simulink model "Realised_inverter_EVOcargo"  (R2021b)
settings: Solver=ode23tb  StartTime=0.0  StopTime=0.02  MaxStep=2.5e-7  RelTol=1e-3  EnableMultiTasking=on
libraries: spsVoltageMeasurementLib x10, spsSeriesRLCBranchLib x9, spsCurrentMeasurementLib x8, spsMosfetLib x6, spsMeanLib x2, simulink x2, spsabctodq0Lib x2, slpidlib x1, spsIdealSwitchLib x1, spsPLL3phLib x1, spsThreePhaseBreakerLib x1, spsThreePhaseSourceLib x1
settings Model: SimulationMode=accelerator  Creator=Алексей  LastModifiedBy=nikol
settings SolverCC: ZeroCrossControl=DisableAll  ZeroCrossAlgorithm=Adaptive  AlgebraicLoopSolver=TrustRegion
settings DataIOCC: SaveFormat=Array  SaveOutput=off  SignalLogging=off  DSMLogging=off  SaveTime=off  ReturnWorkspaceOutputs=off
settings OptimizationCC: LifeSpan=inf
settings DebuggingCC: UnderspecifiedInitializationDetection=Classic  MergeDetectMultiDrivingBlocksExec=none  SolverPrmCheckMsg=warning  AllowSymbolicDim=off  SFUnexpectedBacktrackingDiag=warning  SFNoUnconditionalDefaultTransitionDiag=warning  SFExecutionAtInitializationDiag=none  SFMachineParentedDataDiag=warning  ArithmeticOperatorsInVariantConditions=warning
settings HardwareCC: ProdBitPerPointer=32  ProdBitPerSizeT=32  ProdBitPerPtrDiffT=32  ProdLargestAtomicFloat=None  ProdIntDivRoundTo=Undefined  ProdEndianess=Unspecified  ProdWordSize=32  ProdHWDeviceType=32-bit Generic
settings ModelReferenceCC: PropagateSignalLabelsOutOfModel=off
settings SFSimCC: SimUseLocalCustomCode=off  CustomCodeUndefinedFunction=UseInterfaceOnly
settings RTWCC: RTWUseLocalCustomCode=off
settings CodeAppCC: StateflowObjectComments=on
settings GRTTargetCC: TargetLangStandard=C89/C90 (ANSI)  RTWCAPISignals=on  RTWCAPIParams=on
settings ConfigComp: CovMetricSettings=dw  CovSaveCumulativeToWorkspaceVar=on  CovSaveSingleToWorkspaceVar=on  CovExternalEMLEnable=off  CovSFcnEnable=off
settings SimscapeCC: SimscapeNormalizeSystem=off

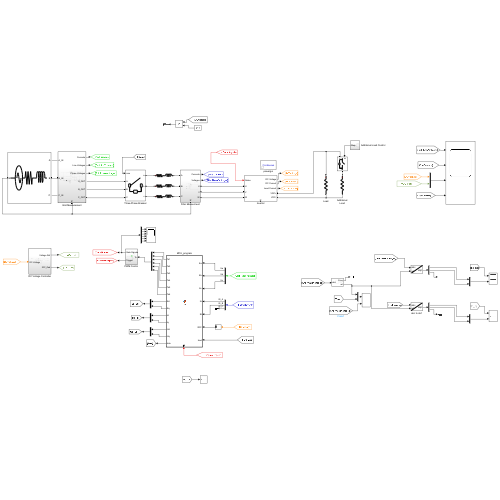
[thumbnail: Simulink's stored preview of the top-level diagram]
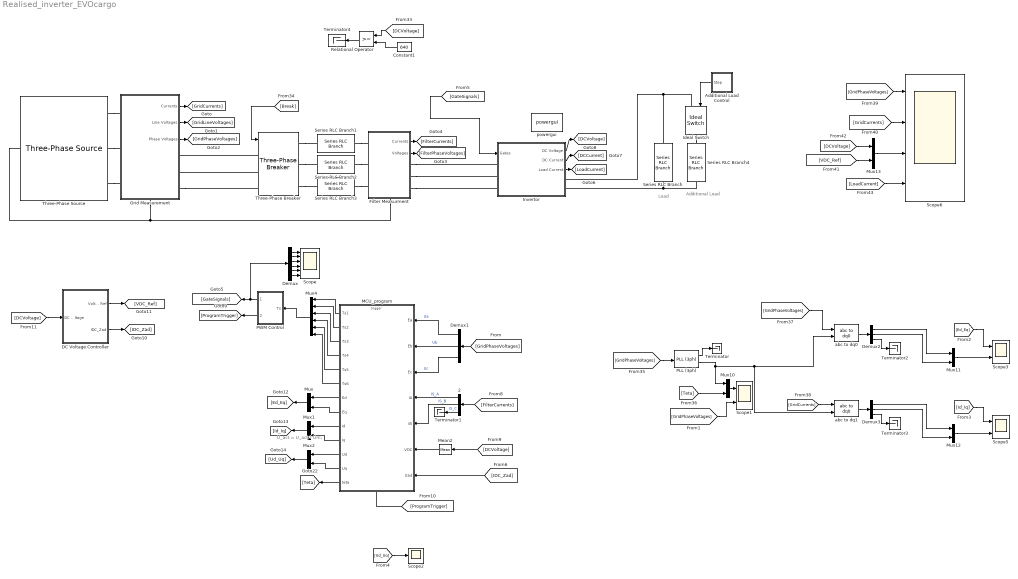
== system Realised_inverter_EVOcargo ==
  note: U_act = U_act * Um;
  note: Load
  note: Additional
      |     Load
  2 : Demux  Outputs=3
  Additional Load Control : Subsystem
  Constant1 : Constant  Value=640
  DC Voltage Controller : Subsystem
  Demux : Demux  Outputs=6
  Demux1 : Demux  Outputs=3
  Demux2 : Demux  Outputs=3
  Demux3 : Demux  Outputs=3
  Filter Measurment : Subsystem
      settings: PortSchema="{\"entries\":[{\"content\":{\"sides\":[{\"content\":{\"connectorIds\":[\"LConn1\",\"LConn2\",\"LConn3\"]},\"type\":\"ConnectorPlacement.EquallySpacedRectSide\",\"uuid\":\"07f1f610-fdaf-45a0-82ba-2fdf13164a36\"},{\"content\":{\"connectorIds\":[\"Out1\",\"Out2\",\"RConn1\",\"RConn2\",\"RConn3\"],\"side\":\"RIGHT\"},\"type\":\"ConnectorPlacement.EquallySpacedRectSide\",\"uuid\":\"0348acf2-7e1d-4672-a4d3-9caea07f27cd\"},{\"content\":{\"connectorIds\":[],\"side\":\"TOP\"},\"type\":\"ConnectorPlacement.EquallySpacedRectSide\",\"uuid\":\"be6f7439-4769-49ea-9688-befff8a6f50f\"},{\"content\":{\"connectorIds\":[\"RConn4\"],\"side\":\"BOTTOM\"},\"type\":\"ConnectorPlacement.EquallySpacedRectSide\",\"uuid\":\"239a5531-0ba1-4f36-bf56-c1872d73e635\"}]},\"type\":\"ConnectorPlacement.EquallySpacedConnector\",\"uuid\":\"325ea333-12da-4f70-8632-c5790302b8cd\"}],\"packageUris\":[\"http://schema.mathworks.com/mf0/Connector/R2020b\"],\"version\":\"1.0\"}"
  Grid Measurement : Subsystem
      settings: PortSchema="{\"entries\":[{\"content\":{\"sides\":[{\"content\":{\"connectorIds\":[\"LConn1\",\"LConn2\",\"LConn3\"]},\"type\":\"ConnectorPlacement.EquallySpacedRectSide\",\"uuid\":\"801c7675-c858-4350-92ae-14638809b1d2\"},{\"content\":{\"connectorIds\":[\"Out1\",\"Out2\",\"Out3\",\"RConn1\",\"RConn2\",\"RConn3\"],\"side\":\"RIGHT\"},\"type\":\"ConnectorPlacement.EquallySpacedRectSide\",\"uuid\":\"0a1e9bc1-9bed-4091-9780-772e4467681a\"},{\"content\":{\"connectorIds\":[],\"side\":\"TOP\"},\"type\":\"ConnectorPlacement.EquallySpacedRectSide\",\"uuid\":\"b82f9080-09d2-46b0-afde-a90803b4583a\"},{\"content\":{\"connectorIds\":[\"RConn4\"],\"side\":\"BOTTOM\"},\"type\":\"ConnectorPlacement.EquallySpacedRectSide\",\"uuid\":\"30cd731b-c919-4dce-85c5-af1a4330ad43\"}]},\"type\":\"ConnectorPlacement.EquallySpacedConnector\",\"uuid\":\"f4513950-4a40-4992-9ffd-40004173624b\"}],\"packageUris\":[\"http://schema.mathworks.com/mf0/Connector/R2020b\"],\"version\":\"1.0\"}"
  Ideal Switch : spsIdealSwitchLib/Ideal Switch  Ron=0.001  Lon=0  IC=0  Rs=1e5  Cs=inf  Measurements=off
  Invertor : Subsystem
      settings: PortSchema="{\"entries\":[{\"content\":{\"sides\":[{\"content\":{\"connectorIds\":[\"In1\",\"LConn1\",\"LConn2\",\"LConn3\"]},\"type\":\"ConnectorPlacement.EquallySpacedRectSide\",\"uuid\":\"92f6c0ba-483d-4b82-8aad-961a4c8cbef5\"},{\"content\":{\"connectorIds\":[\"Out1\",\"Out2\",\"Out3\",\"RConn1\",\"RConn2\"],\"side\":\"RIGHT\"},\"type\":\"ConnectorPlacement.EquallySpacedRectSide\",\"uuid\":\"ef3b9815-5c7f-4cd5-b6c4-990321a57132\"},{\"content\":{\"connectorIds\":[],\"side\":\"TOP\"},\"type\":\"ConnectorPlacement.EquallySpacedRectSide\",\"uuid\":\"4d71fcb3-3c6d-4f29-ac4d-ac71294aa9f2\"},{\"content\":{\"connectorIds\":[\"RConn3\"],\"side\":\"BOTTOM\"},\"type\":\"ConnectorPlacement.EquallySpacedRectSide\",\"uuid\":\"666ddd4c-3a12-4b0d-9e0a-750b3bb002db\"}]},\"type\":\"ConnectorPlacement.EquallySpacedConnector\",\"uuid\":\"7f816b13-2215-4e2c-95a7-fc33abc29cf3\"}],\"packageUris\":[\"http://schema.mathworks.com/mf0/Connector/R2020b\"],\"version\":\"1.0\"}"
  MCU_program : MATLAB Function  TreatAsAtomicUnit=on
  Mean2 : spsMeanLib/Mean  Freq=20000  Vinit=540  Ts=0
  Mux{,1..2,10..13} (7 alike) : Mux  Inputs=2
  Mux4 : Mux  Inputs=6
  PLL (3ph) : spsPLL3phLib/PLL (3ph)  Fmin=45  Par_Init=[0, 50]  ParK=[180, 3200, 1]  TcD=1e-4  MaxRateChangeFreq=12  FilterCutOffFreq=25  Ts=0  AGC=on
  PWM Control : Subsystem
      settings: PortSchema="{\"entries\":[{\"content\":{\"sides\":[{\"content\":{\"connectorIds\":[\"Out1\",\"Out2\"]},\"type\":\"ConnectorPlacement.EquallySpacedRectSide\",\"uuid\":\"d8b25c18-834a-4f60-b770-e16f9b0f8403\"},{\"content\":{\"connectorIds\":[\"In1\"],\"side\":\"RIGHT\"},\"type\":\"ConnectorPlacement.EquallySpacedRectSide\",\"uuid\":\"9dff51bf-dc9f-458e-a11e-8fbf0558d32b\"},{\"content\":{\"connectorIds\":[],\"side\":\"TOP\"},\"type\":\"ConnectorPlacement.EquallySpacedRectSide\",\"uuid\":\"abed77ec-c94b-4080-8d8e-77a9694eba29\"}]},\"type\":\"ConnectorPlacement.EquallySpacedConnector\",\"uuid\":\"310198e6-a417-4af9-8ce6-7d116e9fc291\"}],\"packageUris\":[\"http://schema.mathworks.com/mf0/Connector/R2020b\"],\"version\":\"1.0\"}"
  Relational Operator : RelationalOperator  OutDataTypeStr=boolean  RndMeth=Simplest
  Scope : Scope  NumInputPorts=6
  Scope1 : Scope  NumInputPorts=2
  Scope2 : Scope
  Scope3 : Scope  NumInputPorts=2
  Scope5 : Scope  NumInputPorts=2
  Scope6 : Scope  NumInputPorts=4
  Series RLC Branch : spsSeriesRLCBranchLib/Series RLC Branch  LConnTagsString=__new0  RConnTagsString=__new0  BranchType=R  Resistance=25  Inductance=1e-3  SetiL0=off  InitialCurrent=0  Capacitance=1e-6  Setx0=off  InitialVoltage=0  Measurements=None
  Series RLC Branch1 : spsSeriesRLCBranchLib/Series RLC Branch  LConnTagsString=__new0  RConnTagsString=__new0  BranchType=RL  Resistance=1e-3  Inductance=200e-6  SetiL0=off  InitialCurrent=0  Capacitance=1e-6  Setx0=off  InitialVoltage=0  Measurements=None
  Series RLC Branch2 : spsSeriesRLCBranchLib/Series RLC Branch  LConnTagsString=__new0  RConnTagsString=__new0  BranchType=RL  Resistance=1e-3  Inductance=200e-6  SetiL0=off  InitialCurrent=0  Capacitance=1e-6  Setx0=off  InitialVoltage=0  Measurements=None
  Series RLC Branch3 : spsSeriesRLCBranchLib/Series RLC Branch  LConnTagsString=__new0  RConnTagsString=__new0  BranchType=RL  Resistance=1e-3  Inductance=200e-6  SetiL0=off  InitialCurrent=0  Capacitance=1e-6  Setx0=off  InitialVoltage=0  Measurements=None
  Series RLC Branch4 : spsSeriesRLCBranchLib/Series RLC Branch  LConnTagsString=__new0  RConnTagsString=__new0  BranchType=R  Resistance=25  Inductance=1e-3  SetiL0=off  InitialCurrent=0  Capacitance=1e-6  Setx0=off  InitialVoltage=0  Measurements=None
  Terminator{,1..4} (5 alike) : Terminator
  Three-Phase Breaker : spsThreePhaseBreakerLib/Three-Phase Breaker  InitialState=open  SwitchA=on  SwitchB=on  SwitchC=on  SwitchTimes="[1/60  5/60]"  External=on  BreakerResistance=0.01  SnubberResistance=0.01  SnubberCapacitance=inf  Measurements=None
  Three-Phase Source : spsThreePhaseSourceLib/Three-Phase Source  InternalConnection=Yn  VoltagePhases=on  Voltage=200  PhaseAngle=0  Voltage_phases=[220 220 220]  PhaseAngles_phases=[0 -120 120]  Frequency=50  NonIdealSource=on  SpecifyImpedance=off  Resistance=1e-6  Inductance=30e-9  ShortCircuitLevel=100e6  BaseVoltage=200  XRratio=7  BusType=swing  Pref=10e3  Qref=0  Prefabc=[10e3, 10e3, 10e3]  Qrefabc=[0, 0, 0]  Qmin=-inf  Qmax=inf
  abc to dq0 : spsabctodq0Lib/abc to dq0  Alignment=90 degrees behind phase A axis
  abc to dq1 : spsabctodq0Lib/abc to dq0  Alignment=90 degrees behind phase A axis
  powergui : spspowerguiLib/powergui  Priority=1  SimulationMode=Continuous  SampleTime=50e-6  frequency=60  Iterations=50  frequencyindice=0  Pbase=100e6  ErrMax=1e-4  UnitsV=kV  UnitsW=MW  buscounter=0  FunctionMessages=off  echomessages=off  EnableUseOfTLC=off  CurrentSourceSwitches=on  DisableSnubberDevices=off  DisableRonSwitches=off  DisableVfSwitches=off  DisplayEquations=off  AutomaticDiscreteSolvers=off  SolverType=Tustin  Interpol=off  ExternalGateDelay=off  methode=off  Ts=0  x0status=blocks  SPID=off  SwTol=0  HookPort=off  NonlinearTolerance=1e-4  nMaxIteration=100  ContinueOnMaxIteration=off  RestoreLinks=warning  ResistiveCurrentMeasurement=off  Frange=[0:2:500]  Ylog=off  Xlog=on  ShowGrid=off  save=off  variable=ZData  structure=SD2  ZoomFFT=on  StartTime=0.7  cycles=10  DisplayStyle=4  fundamental=382  FreqAxis=off  MaxFrequency=50000  frequencyindicesteady=1  RmsSteady=1  display=off
  wires:
  MCU_program/6(Ts6) -> Mux4/6
  MCU_program/5(Ts5) -> Mux4/5
  MCU_program/4(Ts4) -> Mux4/4
  MCU_program/3(Ts3) -> Mux4/3
  MCU_program/1(Ts1) -> Mux4/1
  MCU_program/2(Ts2) -> Mux4/2
  Demux1/1 -> MCU_program/1(Ea)  "Ua"
  Demux1/2 -> MCU_program/2(Eb)  "Ub"
  Demux1/3 -> MCU_program/3(Ec)  "Uc"
  Grid Measurement/1(Currents) -> [GridCurrents]
  Grid Measurement/2(Line Voltages) -> [GridLineVoltages]
  Grid Measurement/3(Phase Voltages) -> [GridPhaseVoltages]
  [GridPhaseVoltages] -> Demux1/1
  Filter Measurment/2(Voltages) -> [FilterPhaseVoltages]
  Filter Measurment/1(Currents) -> [FilterCurrents]
  [GateSignals] -> Invertor/1(Gates)
  Additional Load Control/1(Step) -> Ideal Switch/1
  Invertor/3(Load Current) -> [LoadCurrent]
  Invertor/1(DC Voltage) -> [DCVoltage]
  Invertor/2(DC Current) -> [DCCurrent]
  [FilterCurrents] -> 2/1
  2/3 -> Terminator1/1  "IS_C"
  2/1 -> MCU_program/4(IA)  "IS_A"
  2/2 -> MCU_program/5(IB)  "IS_B"
  [DCVoltage] -> Mean2/1
  Mean2/1 -> MCU_program/6(VDC)
  [ProgramTrigger] -> MCU_program/Trigger
  Mux4/1 -> PWM Control/1(Ts)
  PWM Control/1(Gate Signals) -> Demux/1, [GateSignals]
  PWM Control/2(Trigger) -> [ProgramTrigger]
  [DCVoltage] -> DC Voltage Controller/1(DC Voltage)
  DC Voltage Controller/2(IDC_Zad) -> [IDC_Zad]
  [IDC_Zad] -> MCU_program/7(Izad)
  DC Voltage Controller/1(Voltage Ref) -> [VDC_Ref]
  [GridPhaseVoltages] -> PLL (3ph)/1
  PLL (3ph)/1 -> Terminator/1
  PLL (3ph)/2 -> abc to dq0/2, abc to dq1/2, Mux10/1
  [Teta] -> Mux10/2
  [GridPhaseVoltages] -> abc to dq0/1
  abc to dq0/1 -> Demux2/1
  Demux2/3 -> Terminator2/1
  Mux11/1 -> Scope3/2
  Demux2/1 -> Mux11/1
  Demux2/2 -> Mux11/2
  [GridCurrents] -> abc to dq1/1
  Mux12/1 -> Scope5/2
  abc to dq1/1 -> Demux3/1
  Demux3/2 -> Mux12/2
  Demux3/3 -> Terminator3/1
  Demux3/1 -> Mux12/1
  [GridPhaseVoltages] -> Scope6/1
  [GridCurrents] -> Scope6/2
  [DCVoltage] -> Mux13/1
  [VDC_Ref] -> Mux13/2
  Mux13/1 -> Scope6/3
  [LoadCurrent] -> Scope6/4
  [DCVoltage] -> Relational Operator/1
  Constant1/1 -> Relational Operator/2
  Relational Operator/1 -> Terminator4/1
  [Break] -> Three-Phase Breaker/1
  Demux/1 -> Scope/1
  Demux/2 -> Scope/2
  Demux/3 -> Scope/3
  Demux/4 -> Scope/4
  Demux/5 -> Scope/5
  Demux/6 -> Scope/6
  MCU_program/13(teta) -> [Teta]
  Mux10/1 -> Scope1/1
  [GridPhaseVoltages] -> Scope1/2
  MCU_program/7(Ed) -> Mux/1
  MCU_program/8(Eq) -> Mux/2
  MCU_program/9(Id) -> Mux1/1
  MCU_program/10(Iq) -> Mux1/2
  Mux/1 -> [Ed_Eq]
  Mux1/1 -> [Id_Iq]
  [Ed_Eq] -> Scope3/1
  [Id_Iq] -> Scope5/1
  MCU_program/11(Ud) -> Mux2/1
  MCU_program/12(Uq) -> Mux2/2
  Mux2/1 -> [Ud_Uq]
  [Ud_Uq] -> Scope2/1
  connections:
  Ideal Switch/LConn1 -- Invertor/RConn1 -- Series RLC Branch/LConn1
  Series RLC Branch/RConn1 -- Series RLC Branch4/RConn1 -- Invertor/RConn2
  Three-Phase Source/RConn1 -- Grid Measurement/LConn1
  Series RLC Branch2/RConn1 -- Filter Measurment/LConn2
  Three-Phase Source/RConn2 -- Grid Measurement/LConn2
  Three-Phase Source/RConn3 -- Grid Measurement/LConn3
  Series RLC Branch3/RConn1 -- Filter Measurment/LConn3
  Series RLC Branch1/RConn1 -- Filter Measurment/LConn1
  Three-Phase Breaker/LConn2 -- Grid Measurement/RConn2
  Ideal Switch/RConn1 -- Series RLC Branch4/LConn1
  Three-Phase Breaker/LConn1 -- Grid Measurement/RConn1
  Grid Measurement/RConn3 -- Three-Phase Breaker/LConn3
  Filter Measurment/RConn1 -- Invertor/LConn1
  Filter Measurment/RConn2 -- Invertor/LConn2
  Filter Measurment/RConn3 -- Invertor/LConn3
  Filter Measurment/RConn4 -- Three-Phase Source/LConn1 -- Grid Measurement/RConn4
  Three-Phase Breaker/RConn1 -- Series RLC Branch1/LConn1
  Three-Phase Breaker/RConn2 -- Series RLC Branch2/LConn1
  Three-Phase Breaker/RConn3 -- Series RLC Branch3/LConn1

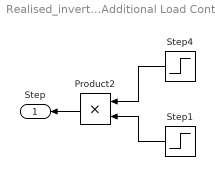
== system Realised_inverter_EVOcargo/Additional Load Control ==
  Product2 : Product
  Step1 : Step  Time=0.15  Before=1  SampleTime=0
  Step4 : Step  Time=0.1  SampleTime=0
  Step : Outport
  wires:
  Step1/1 -> Product2/2
  Step4/1 -> Product2/1
  Product2/1 -> Step/1

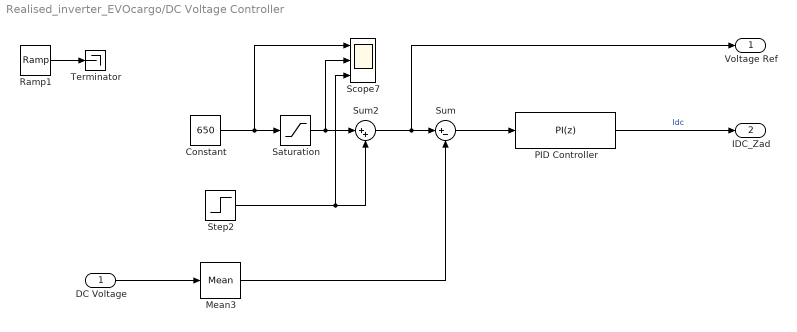
== system Realised_inverter_EVOcargo/DC Voltage Controller ==
  DC Voltage : Inport
  Constant : Constant  Value=650
  Mean3 : spsMeanLib/Mean  Freq=20000  Vinit=540  Ts=0
  PID Controller : slpidlib/PID Controller  Controller=PI  Form=Parallel  TimeDomain=Discrete-time  UseExternalTs=off  SampleTime=20e-6  IntegratorMethod=Forward Euler  FilterMethod=Forward Euler  ControllerParametersSource=internal  P=1  I=150  D=0  UseFilter=on  N=100  TunerSelectOption=Transfer Function Based (PID Tuner App)  ZeroCross=off  InitialConditionSource=internal  InitialConditionForIntegrator=0  InitialConditionForFilter=0  DifferentiatorICPrevScaledInput=0  ExternalReset=none  TrackingMode=off  Kt=1  LimitOutput=on  SatLimitsSource=internal  UpperSaturationLimit=52  LowerSaturationLimit=-52  LinearizeAsGain=on  AntiWindupMode=clamping  Kb=1  POutMin=[]  POutMax=[]  IOutMin=[]  IOutMax=[]  DOutMin=[]  DOutMax=[]  NOutMin=[]  NOutMax=[]  SumOutMin=[]  SumOutMax=[]  SaturationOutMin=[]  SaturationOutMax=[]  PParamMin=[]  PParamMax=[]  IParamMin=[]  IParamMax=[]  DParamMin=[]  DParamMax=[]  NParamMin=[]  NParamMax=[]  KbParamMin=[]  KbParamMax=[]  KtParamMin=[]  KtParamMax=[]  KbOutMin=[]  KbOutMax=[]  KtOutMin=[]  KtOutMax=[]  IntegratorOutMin=[]  IntegratorOutMax=[]  FilterOutMin=[]  FilterOutMax=[]  SumI1OutMin=[]  SumI1OutMax=[]  SumI2OutMin=[]  SumI2OutMax=[]  SumI3OutMin=[]  SumI3OutMax=[]  SumI4OutMin=[]  SumI4OutMax=[]  SumDOutMin=[]  SumDOutMax=[]  DifferentiatorOutMin=[]  DifferentiatorOutMax=[]  FilterDiffOutCoefMin=[]  FilterDiffOutCoefMax=[]  ReciprocalOutMin=[]  ReciprocalOutMax=[]  SumDenOutMin=[]  SumDenOutMax=[]  SumNumOutMin=[]  SumNumOutMax=[]  DivideOutMin=[]  DivideOutMax=[]  UdiffTsProdOutMin=[]  UdiffTsProdOutMax=[]  NTsProdOutMin=[]  NTsProdOutMax=[]  UintegralTsProdOutMin=[]  UintegralTsProdOutMax=[]  UngainTsProdOutMin=[]  UngainTsProdOutMax=[]  IntegratorContinuousStateAttributes=''  IntegratorStateMustResolveToSignalObject=off  IntegratorRTWStateStorageClass=Auto  FilterContinuousStateAttributes=''  FilterStateMustResolveToSignalObject=off  FilterRTWStateStorageClass=Auto  ParallelPVariant=InternalParameters  IdealPVariant=Disabled  IVariant=InternalParameters  DVariant=Disabled  IntegratorVariant=Discrete  SatVariant=Enabled  AWVariant=DiscClampingParallel  PCopyVariant=Disabled  TRVariant=Disabled  FdbkBlocksVariant=Forward  IdealPFdbkVariant=Disabled  SatFdbkVariant=Disabled  DerivativeFilterVariant=Disabled  NVariant=Disabled  NCopyVariant=Disabled_SignalSpec  FilterICVariant=Disabled  IntegratorICVariant=InternalICs  ExternalResetVariant=Disabled  TRSumVariant=Passthrough  SumFdbkVariant=Disabled  SumVariant=Sum_PI  TsampFilterVariant=InternalTs  TsampNgainVariant=Passthrough  TsampIntegralVariant=Passthrough  ExternalSaturationOutDataTypeStr=Inherit: Same as second input
  Ramp1 : simulink/Sources/Ramp  slope=2250  start=0  InitialOutput=540
  Saturation : Saturate  UpperLimit=650  LowerLimit=540
  Scope7 : Scope  NumInputPorts=3
  Step2 : Step  Time=0.2  After=100  SampleTime=0
  Sum : Sum  Inputs=|+-
  Sum2 : Sum  Inputs=|++
  Terminator : Terminator
  Voltage Ref : Outport
  IDC_Zad : Outport  Port=2
  wires:
  Saturation/1 -> Scope7/2, Sum2/1
  Sum2/1 -> Voltage Ref/1, Sum/1
  Constant/1 -> Scope7/1, Saturation/1
  Sum/1 -> PID Controller/1
  PID Controller/1 -> IDC_Zad/1  "Idc"
  Mean3/1 -> Sum/2
  Step2/1 -> Scope7/3, Sum2/2
  DC Voltage/1 -> Mean3/1
  Ramp1/1 -> Terminator/1

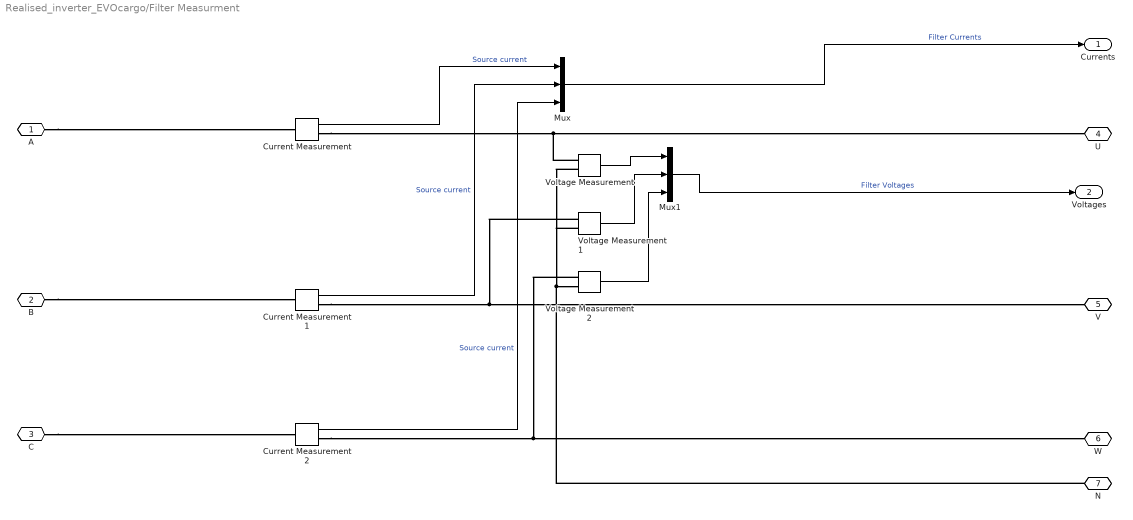
== system Realised_inverter_EVOcargo/Filter Measurment ==
  Current Measurement : spsCurrentMeasurementLib/Current Measurement  PhasorSimulation=off  OutputType=Complex  PSBequivalent=0
  Current Measurement1 : spsCurrentMeasurementLib/Current Measurement  PhasorSimulation=off  OutputType=Complex  PSBequivalent=0
  Current Measurement2 : spsCurrentMeasurementLib/Current Measurement  PhasorSimulation=off  OutputType=Complex  PSBequivalent=0
  Mux : Mux  Inputs=3
  Mux1 : Mux  Inputs=3
  Voltage Measurement : spsVoltageMeasurementLib/Voltage Measurement  PhasorSimulation=off  OutputType=Complex  PSBequivalent=0
  Voltage Measurement1 : spsVoltageMeasurementLib/Voltage Measurement  PhasorSimulation=off  OutputType=Complex  PSBequivalent=0
  Voltage Measurement2 : spsVoltageMeasurementLib/Voltage Measurement  PhasorSimulation=off  OutputType=Complex  PSBequivalent=0
  A : PMIOPort  Side=Left
  B : PMIOPort  Port=2  Side=Left
  C : PMIOPort  Port=3  Side=Left
  U : PMIOPort  Port=4  Side=Right
  V : PMIOPort  Port=5  Side=Right
  W : PMIOPort  Port=6  Side=Right
  N : PMIOPort  Port=7  Side=Right
  Currents : Outport
  Voltages : Outport  Port=2
  wires:
  Current Measurement/1 -> Mux/1  "Source current"
  Mux/1 -> Currents/1  "Filter Currents"
  Current Measurement1/1 -> Mux/2  "Source current"
  Current Measurement2/1 -> Mux/3  "Source current"
  Mux1/1 -> Voltages/1  "Filter Voltages"
  Voltage Measurement/1 -> Mux1/1
  Voltage Measurement1/1 -> Mux1/2
  Voltage Measurement2/1 -> Mux1/3
  connections:
  B/RConn1 -- Current Measurement1/LConn1
  C/RConn1 -- Current Measurement2/LConn1
  Current Measurement2/RConn1 -- Voltage Measurement2/LConn1 -- W/RConn1
  Current Measurement/RConn1 -- Voltage Measurement/LConn1 -- U/RConn1
  Current Measurement1/RConn1 -- Voltage Measurement1/LConn1 -- V/RConn1
  A/RConn1 -- Current Measurement/LConn1
  N/RConn1 -- Voltage Measurement/LConn2 -- Voltage Measurement1/LConn2 -- Voltage Measurement2/LConn2

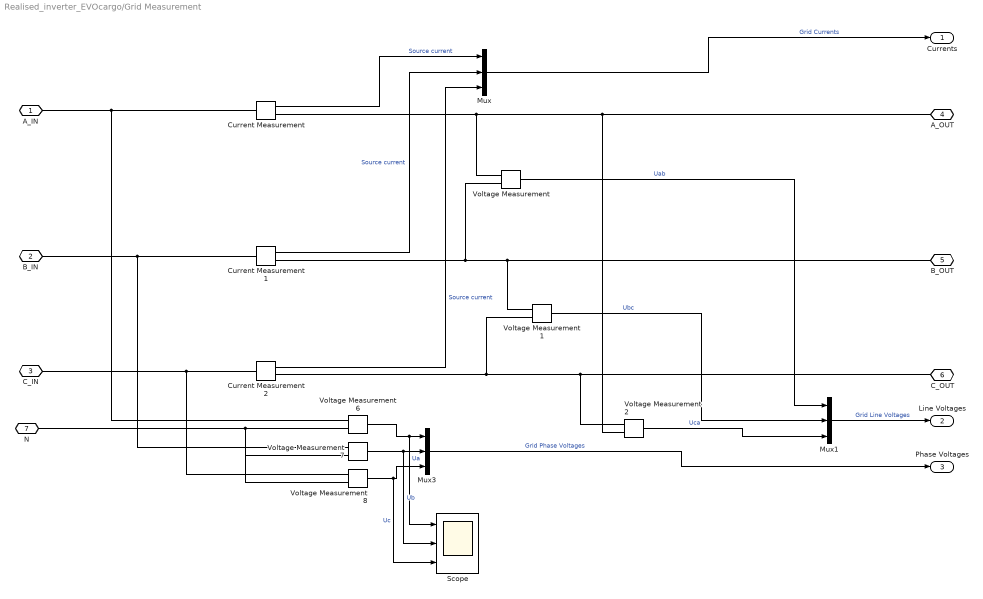
== system Realised_inverter_EVOcargo/Grid Measurement ==
  Current Measurement : spsCurrentMeasurementLib/Current Measurement  PhasorSimulation=off  OutputType=Complex  PSBequivalent=0
  Current Measurement1 : spsCurrentMeasurementLib/Current Measurement  PhasorSimulation=off  OutputType=Complex  PSBequivalent=0
  Current Measurement2 : spsCurrentMeasurementLib/Current Measurement  PhasorSimulation=off  OutputType=Complex  PSBequivalent=0
  Mux : Mux  Inputs=3
  Mux1 : Mux  Inputs=3
  Mux3 : Mux  Inputs=3
  Scope : Scope  NumInputPorts=3
  Voltage Measurement{,1..2,6..8} (6 alike) : spsVoltageMeasurementLib/Voltage Measurement  PhasorSimulation=off  OutputType=Complex  PSBequivalent=0
  A_IN : PMIOPort  Side=Left
  B_IN : PMIOPort  Port=2  Side=Left
  C_IN : PMIOPort  Port=3  Side=Left
  A_OUT : PMIOPort  Port=4  Side=Right
  B_OUT : PMIOPort  Port=5  Side=Right
  C_OUT : PMIOPort  Port=6  Side=Right
  N : PMIOPort  Port=7  Side=Right
  Currents : Outport
  Line Voltages : Outport  Port=2
  Phase Voltages : Outport  Port=3
  wires:
  Current Measurement2/1 -> Mux/3  "Source current"
  Current Measurement1/1 -> Mux/2  "Source current"
  Voltage Measurement1/1 -> Mux1/2  "Ubc"
  Voltage Measurement2/1 -> Mux1/3  "Uca"
  Mux/1 -> Currents/1  "Grid Currents"
  Voltage Measurement/1 -> Mux1/1  "Uab"
  Current Measurement/1 -> Mux/1  "Source current"
  Mux1/1 -> Line Voltages/1  "Grid Line Voltages"
  Mux3/1 -> Phase Voltages/1  "Grid Phase Voltages"
  Voltage Measurement8/1 -> Scope/3, Mux3/3  "Uc"
  Voltage Measurement6/1 -> Scope/1, Mux3/1  "Ua"
  Voltage Measurement7/1 -> Scope/2, Mux3/2  "Ub"
  connections:
  A_IN/RConn1 -- Voltage Measurement6/LConn1 -- Current Measurement/LConn1
  Current Measurement1/RConn1 -- Voltage Measurement/LConn2 -- B_OUT/RConn1 -- Voltage Measurement1/LConn1
  Current Measurement/RConn1 -- Voltage Measurement/LConn1 -- Voltage Measurement2/LConn2 -- A_OUT/RConn1
  Current Measurement2/RConn1 -- Voltage Measurement2/LConn1 -- C_OUT/RConn1 -- Voltage Measurement1/LConn2
  Voltage Measurement6/LConn2 -- Voltage Measurement8/LConn2 -- Voltage Measurement7/LConn2 -- N/RConn1
  C_IN/RConn1 -- Voltage Measurement8/LConn1 -- Current Measurement2/LConn1
  B_IN/RConn1 -- Voltage Measurement7/LConn1 -- Current Measurement1/LConn1

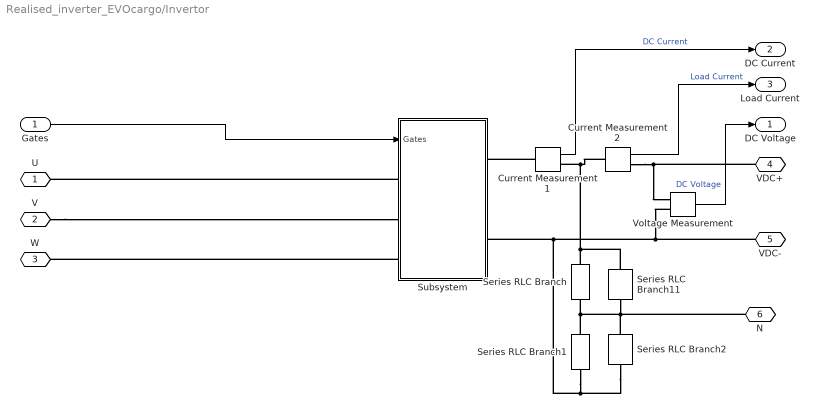
== system Realised_inverter_EVOcargo/Invertor ==
  Gates : Inport
  Current Measurement1 : spsCurrentMeasurementLib/Current Measurement  PhasorSimulation=off  OutputType=Complex  PSBequivalent=0
  Current Measurement2 : spsCurrentMeasurementLib/Current Measurement  PhasorSimulation=off  OutputType=Complex  PSBequivalent=0
  Series RLC Branch : spsSeriesRLCBranchLib/Series RLC Branch  LConnTagsString=__new0  RConnTagsString=__new0  BranchType=C  Resistance=1  Inductance=1e-3  SetiL0=off  InitialCurrent=0  Capacitance=100e-6  Setx0=off  InitialVoltage=280  Measurements=None
  Series RLC Branch1 : spsSeriesRLCBranchLib/Series RLC Branch  LConnTagsString=__new0  RConnTagsString=__new0  BranchType=C  Resistance=1  Inductance=1e-3  SetiL0=off  InitialCurrent=0  Capacitance=100e-6  Setx0=off  InitialVoltage=280  Measurements=None
  Series RLC Branch11 : spsSeriesRLCBranchLib/Series RLC Branch  LConnTagsString=__new0  RConnTagsString=__new0  BranchType=R  Resistance=1e6  Inductance=750e-6  SetiL0=off  InitialCurrent=0  Capacitance=2e-18  Setx0=off  InitialVoltage=0  Measurements=None
  Series RLC Branch2 : spsSeriesRLCBranchLib/Series RLC Branch  LConnTagsString=__new0  RConnTagsString=__new0  BranchType=R  Resistance=1e6  Inductance=750e-6  SetiL0=off  InitialCurrent=0  Capacitance=2e-18  Setx0=off  InitialVoltage=0  Measurements=None
  Subsystem : Subsystem
  Voltage Measurement : spsVoltageMeasurementLib/Voltage Measurement  PhasorSimulation=off  OutputType=Complex  PSBequivalent=0
  U : PMIOPort  Side=Left
  V : PMIOPort  Port=2  Side=Left
  W : PMIOPort  Port=3  Side=Left
  VDC+ : PMIOPort  Port=4  Side=Right
  VDC- : PMIOPort  Port=5  Side=Right
  N : PMIOPort  Port=6  Side=Right
  DC Voltage : Outport  VectorParamsAs1DForOutWhenUnconnected=off
  DC Current : Outport  Port=2  VectorParamsAs1DForOutWhenUnconnected=off
  Load Current : Outport  Port=3  VectorParamsAs1DForOutWhenUnconnected=off
  wires:
  Voltage Measurement/1 -> DC Voltage/1  "DC Voltage"
  Gates/1 -> Subsystem/1(Gates)
  Current Measurement1/1 -> DC Current/1  "DC Current"
  Current Measurement2/1 -> Load Current/1  "Load Current"
  connections:
  Current Measurement1/LConn1 -- Subsystem/RConn1
  Voltage Measurement/LConn2 -- Series RLC Branch2/RConn1 -- Series RLC Branch1/RConn1 -- Subsystem/RConn2 -- VDC-/RConn1
  Subsystem/LConn1 -- U/RConn1
  V/RConn1 -- Subsystem/LConn2
  Subsystem/LConn3 -- W/RConn1
  VDC+/RConn1 -- Current Measurement2/RConn1 -- Voltage Measurement/LConn1
  Current Measurement2/LConn1 -- Series RLC Branch11/LConn1 -- Series RLC Branch/LConn1 -- Current Measurement1/RConn1
  Series RLC Branch1/LConn1 -- N/RConn1 -- Series RLC Branch2/LConn1 -- Series RLC Branch11/RConn1 -- Series RLC Branch/RConn1

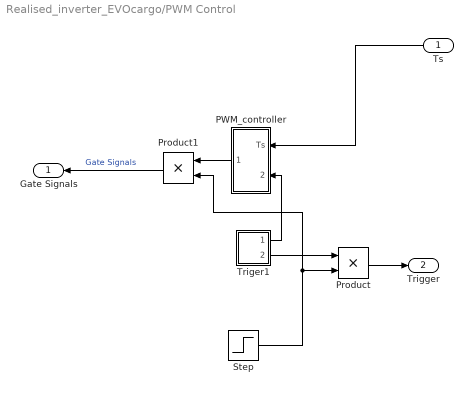
== system Realised_inverter_EVOcargo/PWM Control ==
  Ts : Inport
  PWM_controller : Subsystem
  Product : Product
  Product1 : Product
  Step : Step  Time=0  SampleTime=0
  Triger1 : Subsystem
  Gate Signals : Outport
  Trigger : Outport  Port=2
  wires:
  Triger1/2(2) -> Product/1
  Step/1 -> Product1/2, Product/2
  PWM_controller/1(Tss) -> Product1/1
  Triger1/1(1) -> PWM_controller/2(pila)
  Ts/1 -> PWM_controller/1(Ts)
  Product1/1 -> Gate Signals/1  "Gate Signals"
  Product/1 -> Trigger/1

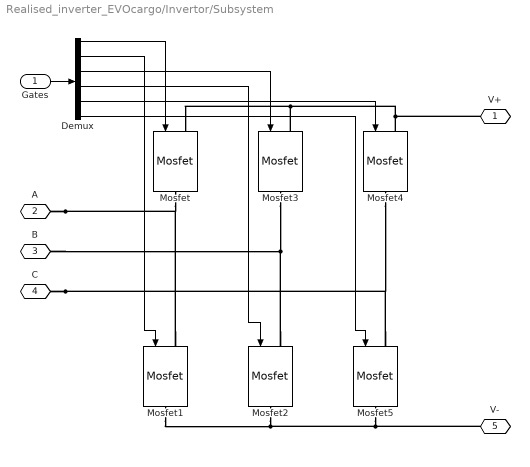
== system Realised_inverter_EVOcargo/Invertor/Subsystem ==
  Gates : Inport
  Demux : Demux  Outputs=6
  Mosfet : spsMosfetLib/Mosfet  Ron=2e-3  Lon=0  Rd=0.01  Vfd=1e-4  IC=0  Rs=1e5  Cs=inf  Measurements=off
  Mosfet{1..5} (5 alike) : spsMosfetLib/Mosfet  Ron=2e-3  Lon=0  Rd=0.01  Vfd=4  IC=0  Rs=1e5  Cs=inf  Measurements=off
  V+ : PMIOPort  Side=Right
  A : PMIOPort  Port=2  Side=Left
  B : PMIOPort  Port=3  Side=Left
  C : PMIOPort  Port=4  Side=Left
  V- : PMIOPort  Port=5  Side=Right
  wires:
  Demux/4 -> Mosfet2/1
  Demux/2 -> Mosfet1/1
  Demux/5 -> Mosfet4/1
  Demux/3 -> Mosfet3/1
  Demux/6 -> Mosfet5/1
  Demux/1 -> Mosfet/1
  Gates/1 -> Demux/1
  connections:
  C/RConn1 -- Mosfet5/LConn1 -- Mosfet4/RConn1
  V-/RConn1 -- Mosfet5/RConn1 -- Mosfet2/RConn1 -- Mosfet1/RConn1
  B/RConn1 -- Mosfet2/LConn1 -- Mosfet3/RConn1
  V+/RConn1 -- Mosfet3/LConn1 -- Mosfet/LConn1 -- Mosfet4/LConn1
  A/RConn1 -- Mosfet/RConn1 -- Mosfet1/LConn1

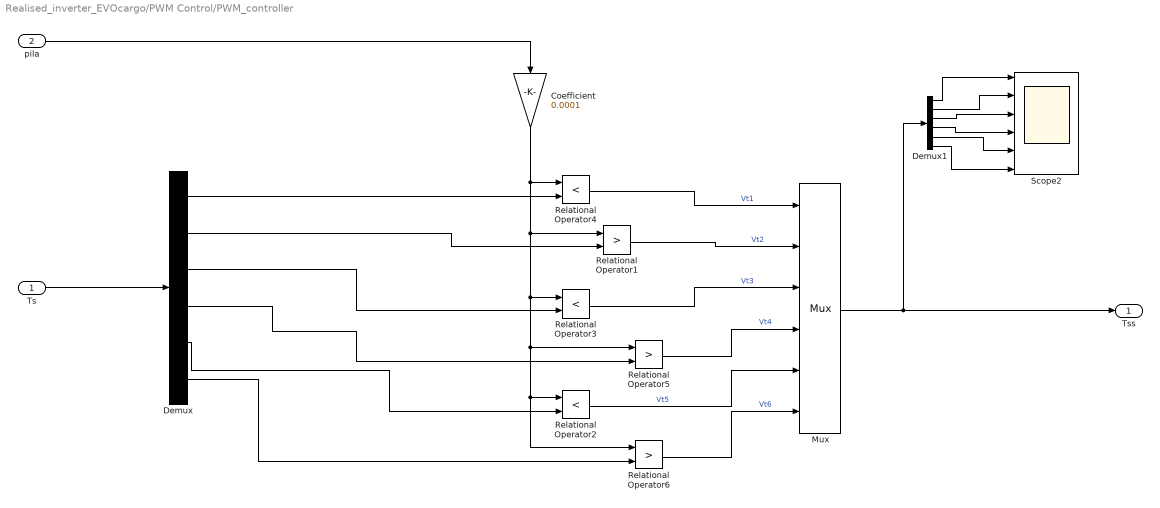
== system Realised_inverter_EVOcargo/PWM Control/PWM_controller ==
  Ts : Inport
  pila : Inport  Port=2
  Coefficient : Gain  Gain=0.0001
  Demux : Demux  Outputs=6
  Demux1 : Demux  Outputs=6
  Mux : Mux  Inputs=6
  Relational Operator1 : RelationalOperator  Operator=>  OutDataTypeStr=boolean  RndMeth=Nearest
  Relational Operator2 : RelationalOperator  Operator=<  OutDataTypeStr=boolean  RndMeth=Nearest
  Relational Operator3 : RelationalOperator  Operator=<  OutDataTypeStr=boolean  RndMeth=Nearest
  Relational Operator4 : RelationalOperator  Operator=<  OutDataTypeStr=boolean  RndMeth=Nearest
  Relational Operator5 : RelationalOperator  Operator=>  OutDataTypeStr=boolean  RndMeth=Nearest
  Relational Operator6 : RelationalOperator  Operator=>  OutDataTypeStr=boolean  RndMeth=Nearest
  Scope2 : Scope  NumInputPorts=6
  Tss : Outport  VectorParamsAs1DForOutWhenUnconnected=off
  wires:
  Relational Operator4/1 -> Mux/1  "Vt1"
  Demux/3 -> Relational Operator3/2
  Demux/5 -> Relational Operator2/2
  Relational Operator3/1 -> Mux/3  "Vt3"
  Relational Operator2/1 -> Mux/5  "Vt5"
  Ts/1 -> Demux/1
  Coefficient/1 -> Relational Operator1/1, Relational Operator3/1, Relational Operator5/1, Relational Operator2/1, Relational Operator6/1, Relational Operator4/1
  Relational Operator1/1 -> Mux/2  "Vt2"
  Relational Operator5/1 -> Mux/4  "Vt4"
  Relational Operator6/1 -> Mux/6  "Vt6"
  Demux/2 -> Relational Operator1/2
  Demux/4 -> Relational Operator5/2
  Demux/6 -> Relational Operator6/2
  Demux/1 -> Relational Operator4/2
  pila/1 -> Coefficient/1
  Mux/1 -> Tss/1, Demux1/1
  Demux1/2 -> Scope2/2
  Demux1/1 -> Scope2/1
  Demux1/4 -> Scope2/4
  Demux1/5 -> Scope2/5
  Demux1/6 -> Scope2/6
  Demux1/3 -> Scope2/3

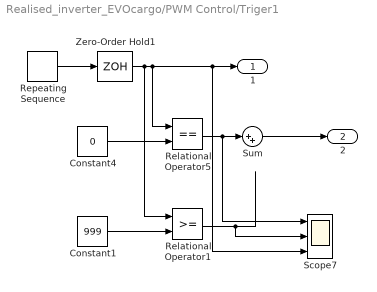
== system Realised_inverter_EVOcargo/PWM Control/Triger1 ==
  Constant1 : Constant  Value=999
  Constant4 : Constant  Value=0
  Relational Operator1 : RelationalOperator  OutDataTypeStr=boolean  RndMeth=Nearest
  Relational Operator5 : RelationalOperator  Operator===  OutDataTypeStr=boolean  RndMeth=Nearest
  Repeating Sequence : simulink/Sources/Repeating Sequence  rep_seq_t=[0 10e-6 20e-6]  rep_seq_y=[0 10000 0]
  Scope7 : Scope  NumInputPorts=3
  Sum : Sum  Inputs=|++
  Zero-Order Hold1 : ZeroOrderHold  SampleTime=2.5e-8
  1 : Outport  VectorParamsAs1DForOutWhenUnconnected=off
  2 : Outport  Port=2  VectorParamsAs1DForOutWhenUnconnected=off
  wires:
  Zero-Order Hold1/1 -> Relational Operator1/1, Relational Operator5/1, Scope7/3, 1/1
  Repeating Sequence/1 -> Zero-Order Hold1/1
  Constant4/1 -> Relational Operator5/2
  Sum/1 -> 2/1
  Constant1/1 -> Relational Operator1/2
  Relational Operator5/1 -> Scope7/1, Sum/1
  Relational Operator1/1 -> Scope7/2

== matlab function Realised_inverter_EVOcargo/MCU_program ==
  data: Ea input; Eb input; Ec input; IA input; IB input; Ts1 output; Ts2 output; Ts3 output; Ts4 output; Ts5 output; Ts6 output; Ed output; Eq output; Id output; Iq output; Ud output; Uq output; VDC input; Izad input; teta output
  events: trigger input RISING_EDGE_EVENT
function [Ts1,Ts2,Ts3,Ts4,Ts5,Ts6, Ed, Eq, Id, Iq, Ud, Uq, teta] = fcn(Ea, Eb, Ec, IA, IB, VDC, Izad)
%время 1/2 ШИМ периода
dt = 20e-6;
R = 1e-3;
L = 200e-6;
wL = 2 * pi * 50 * L;

% RV_Ramp = 0.002;
% 
% persistent RV;
% if isempty(RV)
%     RV = 10;
% end    

dead_time = 1.0;%us
compensate = 0;


kUq_p = 7.5;
kUq_i = kUq_p * R / L;

kUd_p = 7.5;
kUd_i = kUd_p * R / L;


persistent Uq_i;
if isempty(Uq_i)
    Uq_i = 0;
end 
persistent Ud_i;
if isempty(Ud_i)
    Ud_i = 0;
end 

% persistent R_Virtual;
% if isempty(R_Virtual)
%     R_Virtual = 0;
% end    

%Преобразования Кларка Токи
Ialfa = IA;
Ibeta = (2*IB+IA)/sqrt(3);

%Преобразования Кларка Напряжения
Ealfa = Ea;
Ebeta = (Eb - Ec)/sqrt(3);

E_ampl = sqrt(Ealfa^2+Ebeta^2);
teta=acos(Ealfa/E_ampl)*sign(Ebeta)+(sign(Ebeta)-1)*(-pi);

%Преобразование Парка Напряжения
Ed = Ealfa*cos(teta) + Ebeta*sin(teta); 
Eq = Ebeta*cos(teta) - Ealfa*sin(teta); 

%Преобразование Парка Токи 
Id = Ialfa*cos(teta) + Ibeta*sin(teta);
Iq = Ibeta*cos(teta) - Ialfa*sin(teta); 

%ПИ-регулятор для напряжения по оси d
Id_error = Izad - Id;
Ud_p = Id_error * kUd_p;
Ud_i = Ud_i + Id_error * kUd_i * dt;   
%dR = Id * RV;
Ud_pi = Ud_p + Ud_i;% - dR;

Iq_zad = 0;
%ПИ-регулятор для напряжения по оси q
Iq_error = Iq_zad - Iq;
Uq_p = Iq_error * kUq_p;
Uq_i = Uq_i + Iq_error*kUq_i*dt;
%qR = Iq * RV;
Uq_pi  = Uq_p + Uq_i;% - qR;   


% Virtual Resistence Ramp
% RV = RV - (10/RV_Ramp)*dt;
% if RV <= 0;
%     RV = 0;
% end    

Ud = Ed - Ud_pi + Iq * wL;
Uq = Eq - Uq_pi + Id * wL;

Um = (2/3)*VDC/sqrt(Ud^2+Uq^2)*0.95;

if(Um<1)
  Ud = Ud * Um;
  Uq = Uq * Um;
end

%Обратное преобразование Парка
Ua0 = Ud*cos(teta) - Uq*sin(teta);
Ub0 = Ud*sin(teta) + Uq*cos(teta);

vrefa = sqrt(Ua0^2 + Ub0^2);
tetaV = acos(Ua0/vrefa)*sign(Ub0) + (sign(Ub0) - 1)*(-pi);

%алгоритм формирования векторной ШИМ  мертвым веменем dead [мкс]

dead_time = dead_time/(dt*1e6);
a = tetaV;
v2 = vrefa*1.5;
if a >= 0 && a < pi/3 
    n = 1;
elseif  a >= pi/3 && a < 2*pi/3 
    n = 2;
elseif  a >= 2*pi/3 && a < pi 
    n = 3;
elseif  a >= pi && a < 4*pi/3 
    n = 4;
elseif  a >= 4*pi/3 && a < 5*pi/3 
    n = 5;
else 
    n = 6;
end

a_cor = a-(n-1)*pi/3;

T1 = (v2/VDC)*sin(pi/3-a_cor)/sin(pi/3);
T2 = (v2/VDC)*sin(a_cor)/sin(pi/3);
T0 = 1 - T1 - T2;
Ta1 = 0;
Ta3 = 0;
Ta5 = 0; 
switch n
    case 1
        Ta1=T1+T2+T0/2;
        Ta3=T2+T0/2;
        Ta5=T0/2;
    case 2
        Ta1=T1+T0/2;
        Ta3=T1+T2+T0/2;
        Ta5=T0/2;       
    case 3
        Ta1=T0/2;
        Ta3=T1+T2+T0/2;
        Ta5=T2+T0/2;    
    case 4
        Ta1=T0/2;
        Ta3=T1+T0/2;
        Ta5=T1+T2+T0/2;   
    case 5
        Ta1=T2+T0/2;
        Ta3=T0/2;
        Ta5=T1+T2+T0/2;     
    case 6
        Ta1=T1+T2+T0/2;
        Ta3=T0/2;
        Ta5=T1+T0/2;    
end


Ts1 = Ta1 - dead_time/2; 
Ts3 = Ta3 - dead_time/2; 
Ts5 = Ta5 - dead_time/2;
Ts2 = Ta1 + dead_time/2; 
Ts4 = Ta3 + dead_time/2; 
Ts6 = Ta5 + dead_time/2;

if compensate == 1
    if (IA > 0) 
        Ts1 = Ts1 - dead_time/2;
        Ts2 = Ts2 - dead_time/2;
    else
        Ts1 = Ts1 + dead_time/2;
        Ts2 = Ts2 + dead_time/2;           
    end

    if (IB > 0) 
        Ts3 = Ts3 - dead_time/2;
        Ts4 = Ts4 - dead_time/2;
    else
        Ts3 = Ts3 + dead_time/2;
        Ts4 = Ts4 + dead_time/2; 
    end

    if (-(IA+IB) > 0) 
        Ts5 = Ts5 - dead_time/2;
        Ts6 = Ts6 - dead_time/2;
    else
        Ts5 = Ts5 + dead_time/2;
        Ts6 = Ts6 + dead_time/2;           
    end
end

% if(VDC > 1000)
%     Ts1 = 0;
%     Ts2 = 1;
%     Ts3 = 0;
%     Ts4 = 1;
%     Ts5 = 0;
%     Ts6 = 1;
% end

Break = 1;

% if Break == 0
%     Ts1 = 0;
%     Ts2 = 1;
%     Ts3 = 0;
%     Ts4 = 1;
%     Ts5 = 0;
%     Ts6 = 1;
% end

% Ts1 = 0;
% Ts2 = 1;
% Ts3 = 0;
% Ts4 = 1;
% Ts5 = 0;
% Ts6 = 1;

return;
